simulink model "RollControl"  (R2024b)
settings: Solver=VariableStepAuto  StartTime=0.0  StopTime=10  RelTol=1e-3
undefined symbols (not defined in the file or in its folder): Kd, Ki, Kp
libraries: slpidlib x1
settings Model: Creator=Arghya  LastModifiedBy=Arghya

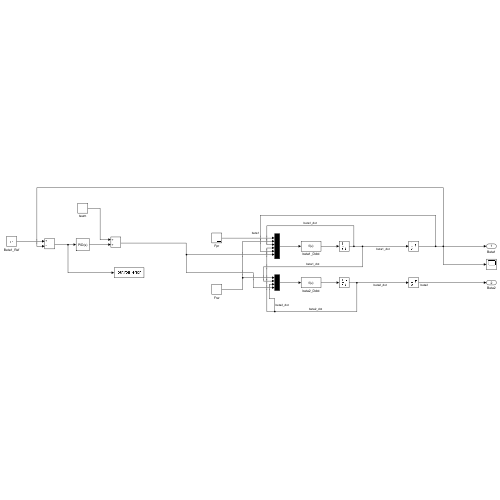
[thumbnail: Simulink's stored preview of the top-level diagram]
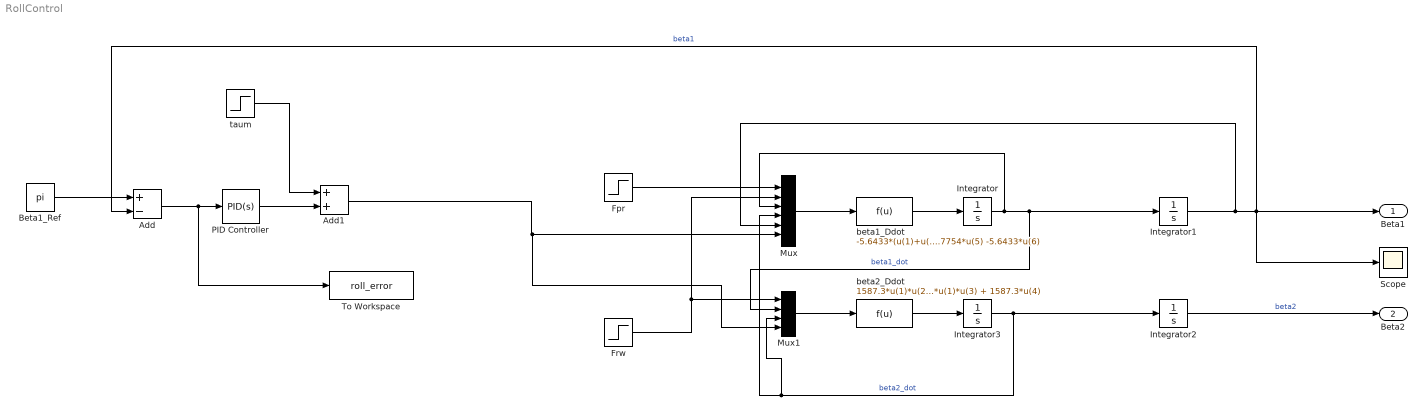
== system RollControl ==
  Add : Sum  Inputs=+-
  Add1 : Sum
  Beta1_Ref : Constant  Value=pi
  Fpr : Step  Before=1  After=0  SampleTime=0.3
  Frw : Step  Before=1  After=0  SampleTime=0.3
  Integrator : Integrator  LimitOutput=on  UpperSaturationLimit=pi/2  LowerSaturationLimit=-pi/2  ContinuousStateAttributes="\"beta1_dot\""
  Integrator1 : Integrator  LimitOutput=on  UpperSaturationLimit=pi/2  LowerSaturationLimit=-pi/2  ContinuousStateAttributes="\"beta1\""
  Integrator2 : Integrator  LimitOutput=on  UpperSaturationLimit=2*pi  LowerSaturationLimit=0  ContinuousStateAttributes="\"beta2\""
  Integrator3 : Integrator  LimitOutput=on  UpperSaturationLimit=2*pi  LowerSaturationLimit=0  ContinuousStateAttributes="\"beta2_dot\""
  Mux : Mux  Inputs=6
  Mux1 : Mux
  PID Controller : slpidlib/PID Controller  Controller=PID  Form=Parallel  TimeDomain=Continuous-time  UseExternalTs=off  SampleTime=-1  IntegratorMethod=Forward Euler  FilterMethod=Forward Euler  ControllerParametersSource=internal  P=Kp  I=Ki  UseKiTs=off  D=Kd  UseExternalDerivativeSource=off  N=100  UseFilter=on  TunerSelectOption=Transfer Function Based (PID Tuner App)  InitialConditionSource=internal  InitialConditionForIntegrator=0  InitialConditionForFilter=0  DifferentiatorICPrevScaledInput=0  ExternalReset=none  TrackingMode=off  Kt=1  LimitOutput=off  SatLimitsSource=internal  UpperSaturationLimit=inf  LowerSaturationLimit=-inf  LinearizeAsGain=on  AntiWindupMode=none  Kb=1  LimitIntegrator=off  UpperIntegratorSaturationLimit=inf  LowerIntegratorSaturationLimit=-inf  POutMin=[]  POutMax=[]  IOutMin=[]  IOutMax=[]  DOutMin=[]  DOutMax=[]  NOutMin=[]  NOutMax=[]  SumOutMin=[]  SumOutMax=[]  SaturationOutMin=[]  SaturationOutMax=[]  PParamMin=[]  PParamMax=[]  IParamMin=[]  IParamMax=[]  DParamMin=[]  DParamMax=[]  NParamMin=[]  NParamMax=[]  KbParamMin=[]  KbParamMax=[]  KtParamMin=[]  KtParamMax=[]  KbOutMin=[]  KbOutMax=[]  KtOutMin=[]  KtOutMax=[]  IntegratorOutMin=[]  IntegratorOutMax=[]  FilterOutMin=[]  FilterOutMax=[]  SumI1OutMin=[]  SumI1OutMax=[]  SumI2OutMin=[]  SumI2OutMax=[]  SumI3OutMin=[]  SumI3OutMax=[]  SumI4OutMin=[]  SumI4OutMax=[]  SumDOutMin=[]  SumDOutMax=[]  DifferentiatorOutMin=[]  DifferentiatorOutMax=[]  FilterDiffOutCoefMin=[]  FilterDiffOutCoefMax=[]  ReciprocalOutMin=[]  ReciprocalOutMax=[]  SumDenOutMin=[]  SumDenOutMax=[]  SumNumOutMin=[]  SumNumOutMax=[]  DivideOutMin=[]  DivideOutMax=[]  UdiffTsProdOutMin=[]  UdiffTsProdOutMax=[]  NTsProdOutMin=[]  NTsProdOutMax=[]  UintegralTsProdOutMin=[]  UintegralTsProdOutMax=[]  UngainTsProdOutMin=[]  UngainTsProdOutMax=[]  ClampingZeroOutDataTypeStr=Inherit: Inherit via back propagation  ClampingZeroOutMin=[]  ClampingZeroOutMax=[]  FilterDenConstantOutDataTypeStr=Inherit: Inherit via back propagation  FilterDenConstantOutMin=[]  FilterDenConstantOutMax=[]  PCopyOutDataTypeStr=Inherit: Inherit via back propagation  PCopyOutMin=[]  PCopyOutMax=[]  NCopyOutDataTypeStr=Inherit: Inherit via back propagation  NCopyOutMin=[]  NCopyOutMax=[]  IntegratorContinuousStateAttributes=''  IntegratorStateMustResolveToSignalObject=off  IntegratorRTWStateStorageClass=Auto  FilterContinuousStateAttributes=''  FilterStateMustResolveToSignalObject=off  FilterRTWStateStorageClass=Auto  ParallelPVariant=InternalParameters  IdealPVariant=Disabled  IVariant=InternalParameters  DVariant=InternalParameters  IntegratorVariant=Continuous  SatVariant=Disabled  AWVariant=Passthrough  PCopyVariant=Disabled  TRVariant=Disabled  FdbkBlocksVariant=Forward  IdealPFdbkVariant=Disabled  SatFdbkVariant=Disabled  DerivativeFilterVariant=ContFilter  NVariant=InternalParameters  NCopyVariant=Disabled  FilterICVariant=InternalICsFilter  IntegratorICVariant=InternalICs  ExternalResetVariant=Disabled  TRSumVariant=Passthrough  SumFdbkVariant=Disabled  SumVariant=Sum_PID  TsampFilterVariant=InternalTs  TsampNgainVariant=Passthrough  TsampIntegralVariant=Disabled_SignalSpec  ExternalSaturationOutDataTypeStr=Inherit: Same as second input  DerivativeSourceVariant=ErrorSignal  PreIntVariant=InternalPreInt
  Scope : Scope
  To Workspace : ToWorkspace  VariableName=roll_error  SampleTime=-1
  beta1_Ddot : Fcn  Expr=-5.6433*(u(1)+u(2))*u(3) + 5.6433*u(4) - 94.7754*u(5) -5.6433*u(6)
  beta2_Ddot : Fcn  Expr=1587.3*u(1)*u(2) - 1587.3*u(1)*u(3) + 1587.3*u(4)
  taum : Step  SampleTime=0
  Beta1 : Outport
  Beta2 : Outport  Port=2
  wires:
  beta1_Ddot/1 -> Integrator/1
  Integrator/1 -> Mux/3, Mux1/2, Integrator1/1  "beta1_dot"
  beta2_Ddot/1 -> Integrator3/1
  Integrator3/1 -> Mux1/3, Mux/4, Integrator2/1  "beta2_dot"
  Integrator1/1 -> Mux/5, Scope/1, Add/2, Beta1/1  "beta1"
  Fpr/1 -> Mux/1
  Frw/1 -> Mux1/1, Mux/2
  Mux/1 -> beta1_Ddot/1
  Mux1/1 -> beta2_Ddot/1
  Add/1 -> To Workspace/1, PID Controller/1
  PID Controller/1 -> Add1/2
  Beta1_Ref/1 -> Add/1
  Integrator2/1 -> Beta2/1  "beta2"
  taum/1 -> Add1/1
  Add1/1 -> Mux1/4, Mux/6
